simulink model "BasicAudio_TranslationEngine64"  (R2022b)
settings: Solver=FixedStepDiscrete  StartTime=0.0  StopTime=5  RelTol=1e-3  EnableMultiTasking=on
InitFcn:
  | % Initialize model
  | run([ ModelRootName() 'Init.m' ]);
  | 
  | % load library data
  | GainLibrary_data;
  | % Load saved values from partition process
  | CapturedConstMask.LoadMapFromFile(bdroot)
model workspace (MAT data in the model file):
  PreampVolumeTable_Idx : Simulink.Signal (value not decoded)
  Range : Simulink.Signal (value not decoded)
  Table_Idx : Simulink.Signal (value not decoded)
undefined symbols (not defined in the file or in its folder): Row
libraries: TuneVar x50, TOP x27, FeaturePath x7, CapturedConstLib x3
(part 3 of 4)

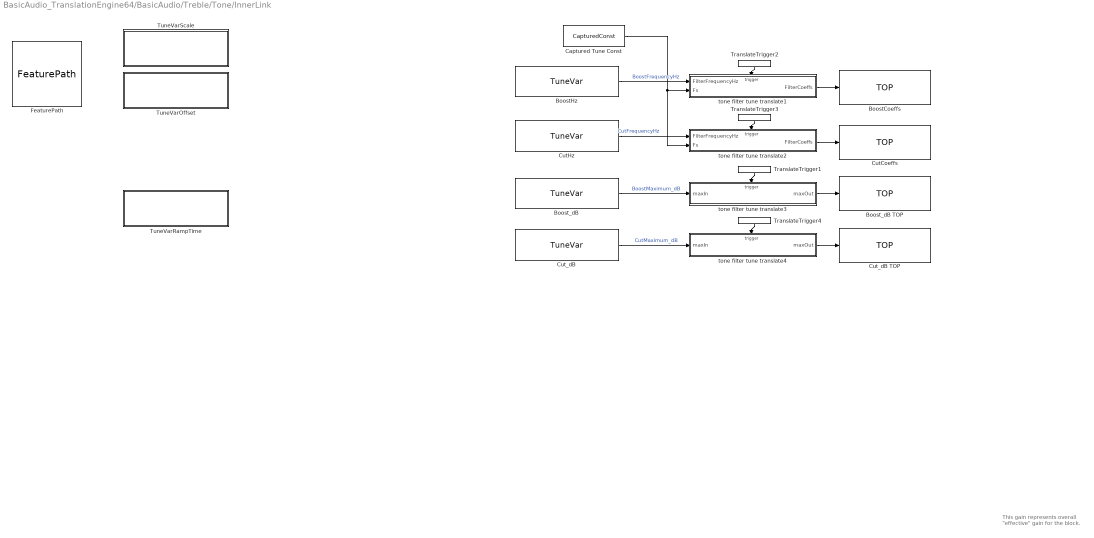
== system BasicAudio_TranslationEngine64/BasicAudio/Treble/Tone/InnerLink ==
  note: This gain represents overall
      | "effective" gain for the block.
  BoostCoeffs : TOP/TOP  TriggerInit=[-490 -218 -340 -162]  TopName=BoostCoeffs  DataTypeOut=single  BankNumber=Config.BankNumber  PreOverlay=false  PostOverlay=false  CompatibilityString=[]  Role=Automatic
      settings: SourceProductName=Bose Talaria
  BoostHz : TuneVar/TuneVar  Description=Indicates the 'corner frequency' of the target frequency band for the 'Boost' filter.  TuneName=BoostFrequencyHz  SpecifyMaxSize=off  VariableDim=1 (Row)  MaxSize=[1 1]  TunabilityNumber=1  MinValue=[]  MaxValue=[]  TriggerInit=[-1025 -225 -855 -175]  MaskValue=Config.DefaultBoostHz
      settings: SourceProductName=Bose Talaria
  Boost_dB : TuneVar/TuneVar  Description=Indicates the maximum impact in dB for the tone boost. This value must be positive. A negative boost impact would imply a gain cut instead!  TuneName=BoostMaximum_dB  SpecifyMaxSize=off  VariableDim=1 (Row)  MaxSize=[1 1]  TunabilityNumber=1  MinValue=[0]  MaxValue=[]  TriggerInit=[-1025 -40 -855 10]  MaskValue=Config.DefaultBoostDb
      settings: SourceProductName=Bose Talaria
  Boost_dB TOP : TOP/TOP  TriggerInit=[-490 -43 -340 13]  TopName=BoostMaximum_dB  DataTypeOut=single  BankNumber=Config.BankNumber  PreOverlay=false  PostOverlay=false  CompatibilityString=[]  Role=Automatic
      settings: SourceProductName=Bose Talaria
  Captured Tune Const : CapturedConstLib/CapturedConst  TriggerInit=[-945 -293 -845 -257]  Role=Automatic
      settings: SourceProductName=Bose Talaria
  CutCoeffs : TOP/TOP  TriggerInit=[-490 -128 -340 -72]  TopName=CutCoeffs  DataTypeOut=single  BankNumber=Config.BankNumber  PreOverlay=false  PostOverlay=false  CompatibilityString=[]  Role=Automatic
      settings: SourceProductName=Bose Talaria
  CutHz : TuneVar/TuneVar  Description=Indicates the 'corner frequency' of the target frequency band for the 'Cut' filter.  TuneName=CutFrequencyHz  SpecifyMaxSize=off  VariableDim=1 (Row)  MaxSize=[1 1]  TunabilityNumber=1  MinValue=[]  MaxValue=[]  TriggerInit=[-1025 -135 -855 -85]  MaskValue=Config.DefaultCutHz
      settings: SourceProductName=Bose Talaria
  Cut_dB : TuneVar/TuneVar  Description=Indicates the maximum impact in dB for the tone cut. This value must be positive. A negative cut impact would imply a gain boost instead!  TuneName=CutMaximum_dB  SpecifyMaxSize=off  VariableDim=1 (Row)  MaxSize=[1 1]  TunabilityNumber=1  MinValue=[0]  MaxValue=[]  TriggerInit=[-1025 45 -855 95]  MaskValue=Config.DefaultCutDb
      settings: SourceProductName=Bose Talaria
  Cut_dB TOP : TOP/TOP  TriggerInit=[-490 42 -340 98]  TopName=CutMaximum_dB  DataTypeOut=single  BankNumber=Config.BankNumber  PreOverlay=false  PostOverlay=false  CompatibilityString=[]  Role=Automatic
      settings: SourceProductName=Bose Talaria
  FeaturePath : FeaturePath/FeaturePath  FeatureName=Treble  IsGroup=off  GroupNumber=-1  IsModule=off  TriggerInit=[-1855 -266 -1740 -159]
      settings: SourceProductName=Bose Talaria
  TranslateTrigger1 : TuneVar/TranslateTrigger  TriggerInit=[-657 -60 -603 -50]
      settings: SourceProductName=Bose Talaria
  TranslateTrigger2 : TuneVar/TranslateTrigger  TriggerInit=[-657 -235 -603 -225]
      settings: SourceProductName=Bose Talaria
  TranslateTrigger3 : TuneVar/TranslateTrigger  TriggerInit=[-657 -145 -603 -135]
      settings: SourceProductName=Bose Talaria
  TranslateTrigger4 : TuneVar/TranslateTrigger  TriggerInit=[-657 25 -603 35]
      settings: SourceProductName=Bose Talaria
  TuneVarOffset : Subsystem  Description=Offset represents the midpoint of the index range, which separates the 'boost' indices from the 'cut' indices.  mask(Talaria Trivial Tune TOP){TriggerInit=[-1670 -213 -1500 -157], TopName=Offset, TuneName=Offset, DataTypeOut=single, MaskValue=Config.DefaultOffset, TunabilityNumber=1, MinValue=[], MaxValue=[], BankNumber=Config.BankNumber, PreOverlay=false, PostOverlay=false, UseSameName=on}
      mask prompts: TriggerInit "Hidden: MoveFcn redraw"; TopName "Name:"; TuneName "Name of TuneVar:"; DataTypeOut "Data type:"; MaskValue "Default Value:"; TunabilityNumber "Tunability:"; MinValue "Min Value:"; MaxValue "Max Value:"; BankNumber "Target memory bank number:"; PreOverlay "Requires pre-overlay action:"; PostOverlay "Requires post-overlay action:"; UseSameName "Use same name for tune variable and TOP"
      mask help: The TuneTOP block encapsultes a Target Overlay Parameter, a Tune Variable, and a Trivial Translation between them.
      mask init:
      | [ok,activeTopPath,activeTunePath] = TuneTOP_Mask.Init(gcbh);
      settings: MoveFcn=TuneTOP_Mask.CB_TriggerInit(gcbh);
      mask Callback TriggerInit: TuneTOP_Mask.CB_TriggerInit(gcbh);
      mask TypeOptions TopName: TOP/TopName
      mask TypeOptions TuneName: Tune Variable/TuneName
      mask TypeOptions DataTypeOut: TOP/DataTypeOut
      mask TypeOptions MaskValue: Tune Variable/MaskValue
      mask TypeOptions TunabilityNumber: Tune Variable/TunabilityNumber
      mask Callback TunabilityNumber: TuneVarMask.CB_TunabilityNumber(gcbh);
      mask TypeOptions MinValue: Tune Variable/MinValue
      mask TypeOptions MaxValue: Tune Variable/MaxValue
      mask TypeOptions BankNumber: TOP/BankNumber
      mask TypeOptions PreOverlay: TOP/PreOverlay
      mask TypeOptions PostOverlay: TOP/PostOverlay
      mask Callback UseSameName: TuneTOP_Mask.CB_UseSameName(gcbh);
      mask DialogControl toolPanel Prompt: Tuning Tool Hints
      mask DialogControl DescriptionGroup Prompt: Description
      mask DialogControl EditDescription Prompt: Edit Description
      mask DialogControl EditDescription Callback: TuneTOP_Mask.CB_EditDescription(gcbh);
      mask DialogControl TunabilityText Prompt: Easy: Changes nearly every tuning.
      mask DialogControl AdvancedPanel Prompt: Advanced
      mask DialogControl ConvertToFullTranslation Prompt: Irreversible conversion to full translation
      mask DialogControl ConvertToFullTranslation Callback: TuneTOP_Mask.CB_ConvertToFullTranslation(gcbh);
      mask DialogControl ErrorContainer Prompt: Error Messages
      mask Display:
      | % retrieve icon definition
      | [path,w,h] = TuneTOP_Mask.Icon();
      | 
      | % retrieve the block's pixel size
      | pos = get(gcbh,'position');
      | bw = pos(3) - pos(1);
      | bh = pos(4) - pos(2);
      | 
      | % draw centered icon
      | xAdj = bw/2 - w/2 + 5;
      | yAdj = bh/2 - h/2 + 4;
      | for i=1:length(path)
      | 	patch(path(i).x+xAdj, path(i).y+yAdj, path(i).rgb);
      | end
      | 
      | % show the top name or an X
      | if (exist('ok','var') && ok)
      | 	text(bw*0.5, bh*0.2, activeTopPath, 'horizontalAlignment', 'center');
      | 	patch(0,0,[1 1 1]);
      | 	patch(bw,bh,[1 1 1]);
      | else
      | 	tx=bw*0.03;
      | 	ty=bh*0.03;
      | 	patch([0 tx bw bw-tx], [ty 0 bh-ty bh], [1 0 0]);
      | 	patch([0 bw-tx bw tx], [bh-ty 0 ty bh], [1 0 0]);
      | end
  TuneVarRampTime : Subsystem  Description=This is the default ramp time that will be used if the RTC message has a '0' for both ramp time and ramp rate.  mask(Talaria Trivial Tune TOP){TriggerInit=[-1670 -18 -1500 38], TopName=ramptime, TuneName=ramptime, DataTypeOut=single, MaskValue=30, TunabilityNumber=1, MinValue=1, MaxValue=100000, BankNumber=0, PreOverlay=false, PostOverlay=false, UseSameName=on}
      mask prompts: TriggerInit "Hidden: MoveFcn redraw"; TopName "Name:"; TuneName "Name of TuneVar:"; DataTypeOut "Data type:"; MaskValue "Default Value:"; TunabilityNumber "Tunability:"; MinValue "Min Value:"; MaxValue "Max Value:"; BankNumber "Target memory bank number:"; PreOverlay "Requires pre-overlay action:"; PostOverlay "Requires post-overlay action:"; UseSameName "Use same name for tune variable and TOP"
      mask help: The TuneTOP block encapsultes a Target Overlay Parameter, a Tune Variable, and a Trivial Translation between them.
      mask init:
      | [ok,activeTopPath,activeTunePath] = TuneTOP_Mask.Init(gcbh);
      settings: MoveFcn=TuneTOP_Mask.CB_TriggerInit(gcbh);
      mask Callback TriggerInit: TuneTOP_Mask.CB_TriggerInit(gcbh);
      mask TypeOptions TopName: TOP/TopName
      mask TypeOptions TuneName: Tune Variable/TuneName
      mask TypeOptions DataTypeOut: TOP/DataTypeOut
      mask TypeOptions MaskValue: Tune Variable/MaskValue
      mask TypeOptions TunabilityNumber: Tune Variable/TunabilityNumber
      mask Callback TunabilityNumber: TuneVarMask.CB_TunabilityNumber(gcbh);
      mask TypeOptions MinValue: Tune Variable/MinValue
      mask TypeOptions MaxValue: Tune Variable/MaxValue
      mask TypeOptions BankNumber: TOP/BankNumber
      mask TypeOptions PreOverlay: TOP/PreOverlay
      mask TypeOptions PostOverlay: TOP/PostOverlay
      mask Callback UseSameName: TuneTOP_Mask.CB_UseSameName(gcbh);
      mask DialogControl toolPanel Prompt: Tuning Tool Hints
      mask DialogControl DescriptionGroup Prompt: Description
      mask DialogControl EditDescription Prompt: Edit Description
      mask DialogControl EditDescription Callback: TuneTOP_Mask.CB_EditDescription(gcbh);
      mask DialogControl TunabilityText Prompt: Easy: Changes nearly every tuning.
      mask DialogControl AdvancedPanel Prompt: Advanced
      mask DialogControl ConvertToFullTranslation Prompt: Irreversible conversion to full translation
      mask DialogControl ConvertToFullTranslation Callback: TuneTOP_Mask.CB_ConvertToFullTranslation(gcbh);
      mask DialogControl ErrorContainer Prompt: Error Messages
      mask Display:
      | % retrieve icon definition
      | [path,w,h] = TuneTOP_Mask.Icon();
      | 
      | % retrieve the block's pixel size
      | pos = get(gcbh,'position');
      | bw = pos(3) - pos(1);
      | bh = pos(4) - pos(2);
      | 
      | % draw centered icon
      | xAdj = bw/2 - w/2 + 5;
      | yAdj = bh/2 - h/2 + 4;
      | for i=1:length(path)
      | 	patch(path(i).x+xAdj, path(i).y+yAdj, path(i).rgb);
      | end
      | 
      | % show the top name or an X
      | if (exist('ok','var') && ok)
      | 	text(bw*0.5, bh*0.2, activeTopPath, 'horizontalAlignment', 'center');
      | 	patch(0,0,[1 1 1]);
      | 	patch(bw,bh,[1 1 1]);
      | else
      | 	tx=bw*0.03;
      | 	ty=bh*0.03;
      | 	patch([0 tx bw bw-tx], [ty 0 bh-ty bh], [1 0 0]);
      | 	patch([0 bw-tx bw tx], [bh-ty 0 ty bh], [1 0 0]);
      | end
  TuneVarScale : Subsystem  Description=Scale is used to normalize the linear gain to a value between +/- 1. The range (0,1] represents a boost while the range [-1,0) represents a cut. We use the number of available indices in each range (mapped to gain values between [-1,1]) as the denominator for normalization, i.e. as the 'Scale'.  mask(Talaria Trivial Tune TOP){TriggerInit=[-1670 -283 -1500 -227], TopName=Scale, TuneName=Scale, DataTypeOut=single, MaskValue=Config.DefaultScale, TunabilityNumber=1, MinValue=[], MaxValue=[], BankNumber=Config.BankNumber, PreOverlay=false, PostOverlay=false, UseSameName=on}
      mask prompts: TriggerInit "Hidden: MoveFcn redraw"; TopName "Name:"; TuneName "Name of TuneVar:"; DataTypeOut "Data type:"; MaskValue "Default Value:"; TunabilityNumber "Tunability:"; MinValue "Min Value:"; MaxValue "Max Value:"; BankNumber "Target memory bank number:"; PreOverlay "Requires pre-overlay action:"; PostOverlay "Requires post-overlay action:"; UseSameName "Use same name for tune variable and TOP"
      mask help: The TuneTOP block encapsultes a Target Overlay Parameter, a Tune Variable, and a Trivial Translation between them.
      mask init:
      | [ok,activeTopPath,activeTunePath] = TuneTOP_Mask.Init(gcbh);
      settings: MoveFcn=TuneTOP_Mask.CB_TriggerInit(gcbh);
      mask Callback TriggerInit: TuneTOP_Mask.CB_TriggerInit(gcbh);
      mask TypeOptions TopName: TOP/TopName
      mask TypeOptions TuneName: Tune Variable/TuneName
      mask TypeOptions DataTypeOut: TOP/DataTypeOut
      mask TypeOptions MaskValue: Tune Variable/MaskValue
      mask TypeOptions TunabilityNumber: Tune Variable/TunabilityNumber
      mask Callback TunabilityNumber: TuneVarMask.CB_TunabilityNumber(gcbh);
      mask TypeOptions MinValue: Tune Variable/MinValue
      mask TypeOptions MaxValue: Tune Variable/MaxValue
      mask TypeOptions BankNumber: TOP/BankNumber
      mask TypeOptions PreOverlay: TOP/PreOverlay
      mask TypeOptions PostOverlay: TOP/PostOverlay
      mask Callback UseSameName: TuneTOP_Mask.CB_UseSameName(gcbh);
      mask DialogControl toolPanel Prompt: Tuning Tool Hints
      mask DialogControl DescriptionGroup Prompt: Description
      mask DialogControl EditDescription Prompt: Edit Description
      mask DialogControl EditDescription Callback: TuneTOP_Mask.CB_EditDescription(gcbh);
      mask DialogControl TunabilityText Prompt: Easy: Changes nearly every tuning.
      mask DialogControl AdvancedPanel Prompt: Advanced
      mask DialogControl ConvertToFullTranslation Prompt: Irreversible conversion to full translation
      mask DialogControl ConvertToFullTranslation Callback: TuneTOP_Mask.CB_ConvertToFullTranslation(gcbh);
      mask DialogControl ErrorContainer Prompt: Error Messages
      mask Display:
      | % retrieve icon definition
      | [path,w,h] = TuneTOP_Mask.Icon();
      | 
      | % retrieve the block's pixel size
      | pos = get(gcbh,'position');
      | bw = pos(3) - pos(1);
      | bh = pos(4) - pos(2);
      | 
      | % draw centered icon
      | xAdj = bw/2 - w/2 + 5;
      | yAdj = bh/2 - h/2 + 4;
      | for i=1:length(path)
      | 	patch(path(i).x+xAdj, path(i).y+yAdj, path(i).rgb);
      | end
      | 
      | % show the top name or an X
      | if (exist('ok','var') && ok)
      | 	text(bw*0.5, bh*0.2, activeTopPath, 'horizontalAlignment', 'center');
      | 	patch(0,0,[1 1 1]);
      | 	patch(bw,bh,[1 1 1]);
      | else
      | 	tx=bw*0.03;
      | 	ty=bh*0.03;
      | 	patch([0 tx bw bw-tx], [ty 0 bh-ty bh], [1 0 0]);
      | 	patch([0 bw-tx bw tx], [bh-ty 0 ty bh], [1 0 0]);
      | end
  tone filter tune translate1 : MATLAB Function  TreatAsAtomicUnit=on  mask{MaskFilterType=Config.FilterType}
      mask prompts: MaskFilterType "Filter type"
  tone filter tune translate2 : MATLAB Function  TreatAsAtomicUnit=on  mask{MaskFilterType=Config.FilterType}
      mask prompts: MaskFilterType "Filter type"
  tone filter tune translate3 : MATLAB Function  TreatAsAtomicUnit=on
  tone filter tune translate4 : MATLAB Function  TreatAsAtomicUnit=on
  wires:
  TranslateTrigger2/1 -> tone filter tune translate1/Trigger
  BoostHz/1 -> tone filter tune translate1/1(FilterFrequencyHz)  "BoostFrequencyHz"
  TranslateTrigger3/1 -> tone filter tune translate2/Trigger
  CutHz/1 -> tone filter tune translate2/1(FilterFrequencyHz)  "CutFrequencyHz"
  tone filter tune translate1/1(FilterCoeffs) -> BoostCoeffs/1
  tone filter tune translate2/1(FilterCoeffs) -> CutCoeffs/1
  Boost_dB/1 -> tone filter tune translate3/1(maxIn)  "BoostMaximum_dB"
  tone filter tune translate3/1(maxOut) -> Boost_dB TOP/1
  Cut_dB/1 -> tone filter tune translate4/1(maxIn)  "CutMaximum_dB"
  tone filter tune translate4/1(maxOut) -> Cut_dB TOP/1
  Captured Tune Const/1 -> tone filter tune translate2/2(Fs), tone filter tune translate1/2(Fs)
  TranslateTrigger1/1 -> tone filter tune translate3/Trigger
  TranslateTrigger4/1 -> tone filter tune translate4/Trigger

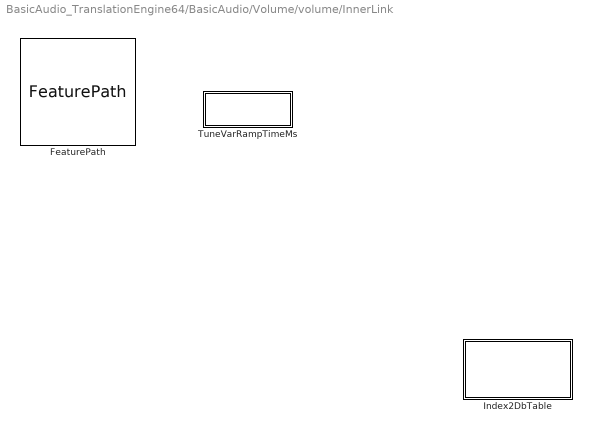
== system BasicAudio_TranslationEngine64/BasicAudio/Volume/volume/InnerLink ==
  FeaturePath : FeaturePath/FeaturePath  FeatureName=Volume  IsGroup=off  GroupNumber=-1  IsModule=off  TriggerInit=[640 269 755 376]
      settings: SourceProductName=Bose Talaria
  Index2DbTable : Subsystem  mask(Blocklib Index2DbTable){Config=Config}
      mask prompts: Config "Index2DbTableConfig"
      mask help: This block contains overlay tuning data for an index-to-dB lookup table. Provide the maximum number of points in the table as a build-time variable. The TuneVar is variable size, but must define at least two points (i.e. two rows, or four values).
      mask init:
      | blkh=gcbh;
      | Config=BTConfig.Assert(blkh,Config);
      | 
      | Config.Validate();
      mask Help:
      | This block contains overlay tuning data which defines an index-to-dB lookup table.
      | Each row of the tuning data contains an index and a dB value.
      | 
      | Tuning data
      | ---------------
      |    tune index: normalized value between 0 and 1
      |    tune value: dB value such as 0 (aka linear "1") or -100 (aka "very quiet")
      | 
      | Inports
      | ----------
      |    trigger: function call trigger that invokes the lookup from inport index to output dB
      |    index: an 8-bit integer index between [0:255] corresponding to the tuning index range [0:1]
      | 
      | Outport
      | -----------
      |    The resulting dB value looked up in the tuned table by using the inbound index
  TuneVarRampTimeMs : Subsystem  mask(Talaria Trivial Tune TOP){TriggerInit=[825 324 910 356], TopName=RampTime, TuneName=RampTime, DataTypeOut=single, MaskValue=100, TunabilityNumber=1, MinValue=[], MaxValue=[], BankNumber=0, PreOverlay=false, PostOverlay=false, UseSameName=on}
      mask prompts: TriggerInit "Hidden: MoveFcn redraw"; TopName "Name:"; TuneName "Name of TuneVar:"; DataTypeOut "Data type:"; MaskValue "Default Value:"; TunabilityNumber "Tunability:"; MinValue "Min Value:"; MaxValue "Max Value:"; BankNumber "Target memory bank number:"; PreOverlay "Requires pre-overlay action:"; PostOverlay "Requires post-overlay action:"; UseSameName "Use same name for tune variable and TOP"
      mask help: The TuneTOP block encapsultes a Target Overlay Parameter, a Tune Variable, and a Trivial Translation between them.
      mask init:
      | [ok,activeTopPath,activeTunePath] = TuneTOP_Mask.Init(gcbh);
      settings: MoveFcn=TuneTOP_Mask.CB_TriggerInit(gcbh);
      mask Callback TriggerInit: TuneTOP_Mask.CB_TriggerInit(gcbh);
      mask TypeOptions TopName: TOP/TopName
      mask TypeOptions TuneName: Tune Variable/TuneName
      mask TypeOptions DataTypeOut: TOP/DataTypeOut
      mask TypeOptions MaskValue: Tune Variable/MaskValue
      mask TypeOptions TunabilityNumber: Tune Variable/TunabilityNumber
      mask Callback TunabilityNumber: TuneVarMask.CB_TunabilityNumber(gcbh);
      mask TypeOptions MinValue: Tune Variable/MinValue
      mask TypeOptions MaxValue: Tune Variable/MaxValue
      mask TypeOptions BankNumber: TOP/BankNumber
      mask TypeOptions PreOverlay: TOP/PreOverlay
      mask TypeOptions PostOverlay: TOP/PostOverlay
      mask Callback UseSameName: TuneTOP_Mask.CB_UseSameName(gcbh);
      mask DialogControl toolPanel Prompt: Tuning Tool Hints
      mask DialogControl DescriptionGroup Prompt: Description
      mask DialogControl EditDescription Prompt: Edit Description
      mask DialogControl EditDescription Callback: TuneTOP_Mask.CB_EditDescription(gcbh);
      mask DialogControl TunabilityText Prompt: Easy: Changes nearly every tuning.
      mask DialogControl AdvancedPanel Prompt: Advanced
      mask DialogControl ConvertToFullTranslation Prompt: Irreversible conversion to full translation
      mask DialogControl ConvertToFullTranslation Callback: TuneTOP_Mask.CB_ConvertToFullTranslation(gcbh);
      mask DialogControl ErrorContainer Prompt: Error Messages
      mask DialogControl ErrorText Prompt: No overlay group found. Declare one in a FeaturePath.
      mask Display:
      | % retrieve icon definition
      | [path,w,h] = TuneTOP_Mask.Icon();
      | 
      | % retrieve the block's pixel size
      | pos = get(gcbh,'position');
      | bw = pos(3) - pos(1);
      | bh = pos(4) - pos(2);
      | 
      | % draw centered icon
      | xAdj = bw/2 - w/2 + 5;
      | yAdj = bh/2 - h/2 + 4;
      | for i=1:length(path)
      | 	patch(path(i).x+xAdj, path(i).y+yAdj, path(i).rgb);
      | end
      | 
      | % show the top name or an X
      | if (exist('ok','var') && ok)
      | 	text(bw*0.5, bh*0.2, activeTopPath, 'horizontalAlignment', 'center');
      | 	patch(0,0,[1 1 1]);
      | 	patch(bw,bh,[1 1 1]);
      | else
      | 	tx=bw*0.03;
      | 	ty=bh*0.03;
      | 	patch([0 tx bw bw-tx], [ty 0 bh-ty bh], [1 0 0]);
      | 	patch([0 bw-tx bw tx], [bh-ty 0 ty bh], [1 0 0]);
      | end

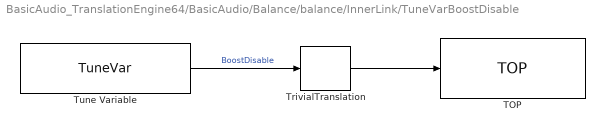
== system BasicAudio_TranslationEngine64/BasicAudio/Balance/balance/InnerLink/TuneVarBoostDisable ==
  TOP : TOP/TOP  TriggerInit=[440 20 585 80]  TopName=BoostDisable  DataTypeOut=single  BankNumber=BankNumber  PreOverlay=PreOverlay  PostOverlay=PostOverlay  CompatibilityString=[]  Role=Automatic
      settings: SourceProductName=Bose Talaria
  TrivialTranslation : TuneVar/TrivialTranslation  TriggerInit=[300 28 350 72]
      settings: SourceProductName=Bose Talaria
  Tune Variable : TuneVar/TuneVar  TuneName=BoostDisable  SpecifyMaxSize=off  VariableDim=1 (Row)  MaxSize=[1 1]  TunabilityNumber=2  MinValue=MinValue  MaxValue=MaxValue  TriggerInit=[20 25 190 75]  MaskValue=MaskValue
      settings: SourceProductName=Bose Talaria
  wires:
  Tune Variable/1 -> TrivialTranslation/1  "BoostDisable"
  TrivialTranslation/1 -> TOP/1

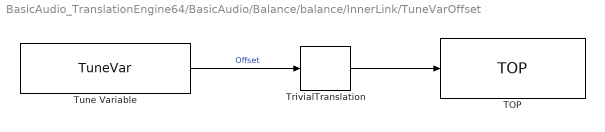
== system BasicAudio_TranslationEngine64/BasicAudio/Balance/balance/InnerLink/TuneVarOffset ==
  TOP : TOP/TOP  TriggerInit=[440 20 585 80]  TopName=Offset  DataTypeOut=single  BankNumber=BankNumber  PreOverlay=PreOverlay  PostOverlay=PostOverlay  CompatibilityString=[]  Role=Automatic
      settings: SourceProductName=Bose Talaria
  TrivialTranslation : TuneVar/TrivialTranslation  TriggerInit=[300 28 350 72]
      settings: SourceProductName=Bose Talaria
  Tune Variable : TuneVar/TuneVar  TuneName=Offset  SpecifyMaxSize=off  VariableDim=1 (Row)  MaxSize=[1 1]  TunabilityNumber=3  MinValue=MinValue  MaxValue=MaxValue  TriggerInit=[20 25 190 75]  MaskValue=MaskValue
      settings: SourceProductName=Bose Talaria
  wires:
  Tune Variable/1 -> TrivialTranslation/1  "Offset"
  TrivialTranslation/1 -> TOP/1

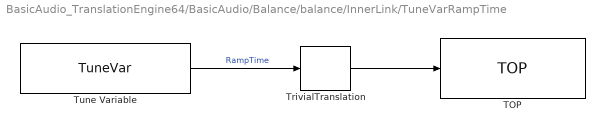
== system BasicAudio_TranslationEngine64/BasicAudio/Balance/balance/InnerLink/TuneVarRampTime ==
  TOP : TOP/TOP  TriggerInit=[440 20 585 80]  TopName=RampTime  DataTypeOut=single  BankNumber=BankNumber  PreOverlay=PreOverlay  PostOverlay=PostOverlay  CompatibilityString=[]  Role=Automatic
      settings: SourceProductName=Bose Talaria
  TrivialTranslation : TuneVar/TrivialTranslation  TriggerInit=[300 28 350 72]
      settings: SourceProductName=Bose Talaria
  Tune Variable : TuneVar/TuneVar  TuneName=RampTime  SpecifyMaxSize=off  VariableDim=1 (Row)  MaxSize=[1 1]  TunabilityNumber=2  MinValue=MinValue  MaxValue=MaxValue  TriggerInit=[20 25 190 75]  MaskValue=MaskValue
      settings: SourceProductName=Bose Talaria
  wires:
  Tune Variable/1 -> TrivialTranslation/1  "RampTime"
  TrivialTranslation/1 -> TOP/1

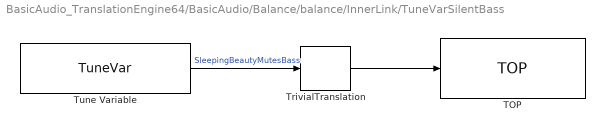
== system BasicAudio_TranslationEngine64/BasicAudio/Balance/balance/InnerLink/TuneVarSilentBass ==
  TOP : TOP/TOP  TriggerInit=[440 20 585 80]  TopName=SleepingBeautyMutesBass  DataTypeOut=single  BankNumber=BankNumber  PreOverlay=PreOverlay  PostOverlay=PostOverlay  CompatibilityString=[]  Role=Automatic
      settings: SourceProductName=Bose Talaria
  TrivialTranslation : TuneVar/TrivialTranslation  TriggerInit=[300 28 350 72]
      settings: SourceProductName=Bose Talaria
  Tune Variable : TuneVar/TuneVar  TuneName=SleepingBeautyMutesBass  SpecifyMaxSize=off  VariableDim=1 (Row)  MaxSize=[1 1]  TunabilityNumber=1  MinValue=MinValue  MaxValue=MaxValue  TriggerInit=[20 25 190 75]  MaskValue=MaskValue
      settings: SourceProductName=Bose Talaria
  wires:
  Tune Variable/1 -> TrivialTranslation/1  "SleepingBeautyMutesBass"
  TrivialTranslation/1 -> TOP/1

== system BasicAudio_TranslationEngine64/BasicAudio/Balance/balance/InnerLink/TuneVarSilentExtreme ==
  TOP : TOP/TOP  TriggerInit=[440 20 585 80]  TopName=EnableSilentExtreme  DataTypeOut=single  BankNumber=BankNumber  PreOverlay=PreOverlay  PostOverlay=PostOverlay  CompatibilityString=[]  Role=Automatic
      settings: SourceProductName=Bose Talaria
  TrivialTranslation : TuneVar/TrivialTranslation  TriggerInit=[300 28 350 72]
      settings: SourceProductName=Bose Talaria
  Tune Variable : TuneVar/TuneVar  TuneName=EnableSilentExtreme  SpecifyMaxSize=off  VariableDim=1 (Row)  MaxSize=[1 1]  TunabilityNumber=2  MinValue=MinValue  MaxValue=MaxValue  TriggerInit=[20 25 190 75]  MaskValue=MaskValue
      settings: SourceProductName=Bose Talaria
  wires:
  Tune Variable/1 -> TrivialTranslation/1  "EnableSilentExtreme"
  TrivialTranslation/1 -> TOP/1

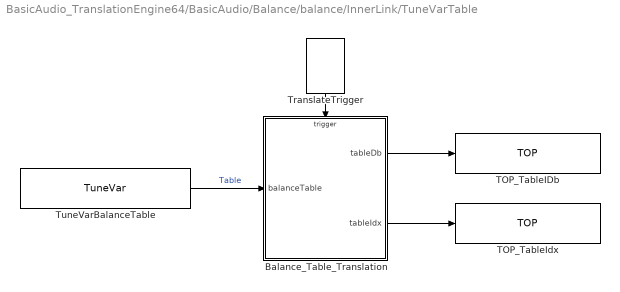
== system BasicAudio_TranslationEngine64/BasicAudio/Balance/balance/InnerLink/TuneVarTable ==
  Balance_Table_Translation : MATLAB Function  TreatAsAtomicUnit=on
  TOP_TableIDb : TOP/TOP  TriggerInit=[455 -5 600 35]  TopName=TableDb  DataTypeOut=single  BankNumber=0  PreOverlay=false  PostOverlay=false  CompatibilityString=[]  Role=Automatic
      settings: SourceProductName=Bose Talaria
  TOP_TableIdx : TOP/TOP  TriggerInit=[455 65 600 105]  TopName=TableIdx  DataTypeOut=single  BankNumber=Config.BankNumber  PreOverlay=false  PostOverlay=false  CompatibilityString=[]  Role=Automatic
      settings: SourceProductName=Bose Talaria
  TranslateTrigger : TuneVar/TranslateTrigger  TriggerInit=[306 -100 344 -45]
      settings: SourceProductName=Bose Talaria
  TuneVarBalanceTable : TuneVar/TuneVar  Description=Define the balance curve using a table, with the first column being the list of indices and the second column being the corresponding balance gains in dB. Gain values for indices in between the elements in the table are linearly interpolated.  TuneName=Table  SpecifyMaxSize=on  VariableDim=1 (Row)  MaxSize=[30 2]  TunabilityNumber=3  MinValue=0  MaxValue=[]  TriggerInit=[20 30 190 70]  MaskValue=[[0,10,31,52,74,95,116,128,138,159,180,202,223,244,255];[-30,-27,-14,-7,-5,-3,-1,0,-1,-3,-5,-7,-14,-27,-30]]'
      settings: SourceProductName=Bose Talaria
  wires:
  Balance_Table_Translation/1(tableDb) -> TOP_TableIDb/1
  TranslateTrigger/1 -> Balance_Table_Translation/Trigger
  Balance_Table_Translation/2(tableIdx) -> TOP_TableIdx/1
  TuneVarBalanceTable/1 -> Balance_Table_Translation/1(balanceTable)  "Table"

== system BasicAudio_TranslationEngine64/BasicAudio/Bass/Tone/InnerLink/TuneVarOffset ==
  TOP : TOP/TOP  TriggerInit=[440 20 585 80]  TopName=Offset  DataTypeOut=single  BankNumber=BankNumber  PreOverlay=PreOverlay  PostOverlay=PostOverlay  CompatibilityString=[]  Role=Automatic
      settings: SourceProductName=Bose Talaria
  TrivialTranslation : TuneVar/TrivialTranslation  TriggerInit=[300 28 350 72]
      settings: SourceProductName=Bose Talaria
  Tune Variable : TuneVar/TuneVar  TuneName=Offset  SpecifyMaxSize=off  VariableDim=1 (Row)  MaxSize=[1 1]  TunabilityNumber=1  MinValue=MinValue  MaxValue=MaxValue  TriggerInit=[20 25 190 75]  MaskValue=MaskValue
      settings: SourceProductName=Bose Talaria
  wires:
  Tune Variable/1 -> TrivialTranslation/1  "Offset"
  TrivialTranslation/1 -> TOP/1

== system BasicAudio_TranslationEngine64/BasicAudio/Bass/Tone/InnerLink/TuneVarRampTime ==
  TOP : TOP/TOP  TriggerInit=[440 20 585 80]  TopName=ramptime  DataTypeOut=single  BankNumber=BankNumber  PreOverlay=PreOverlay  PostOverlay=PostOverlay  CompatibilityString=[]  Role=Automatic
      settings: SourceProductName=Bose Talaria
  TrivialTranslation : TuneVar/TrivialTranslation  TriggerInit=[300 28 350 72]
      settings: SourceProductName=Bose Talaria
  Tune Variable : TuneVar/TuneVar  TuneName=ramptime  SpecifyMaxSize=off  VariableDim=1 (Row)  MaxSize=[1 1]  TunabilityNumber=1  MinValue=MinValue  MaxValue=MaxValue  TriggerInit=[20 25 190 75]  MaskValue=MaskValue
      settings: SourceProductName=Bose Talaria
  wires:
  Tune Variable/1 -> TrivialTranslation/1  "ramptime"
  TrivialTranslation/1 -> TOP/1

== system BasicAudio_TranslationEngine64/BasicAudio/Bass/Tone/InnerLink/TuneVarScale ==
  TOP : TOP/TOP  TriggerInit=[440 20 585 80]  TopName=Scale  DataTypeOut=single  BankNumber=BankNumber  PreOverlay=PreOverlay  PostOverlay=PostOverlay  CompatibilityString=[]  Role=Automatic
      settings: SourceProductName=Bose Talaria
  TrivialTranslation : TuneVar/TrivialTranslation  TriggerInit=[300 28 350 72]
      settings: SourceProductName=Bose Talaria
  Tune Variable : TuneVar/TuneVar  TuneName=Scale  SpecifyMaxSize=off  VariableDim=1 (Row)  MaxSize=[1 1]  TunabilityNumber=1  MinValue=MinValue  MaxValue=MaxValue  TriggerInit=[20 25 190 75]  MaskValue=MaskValue
      settings: SourceProductName=Bose Talaria
  wires:
  Tune Variable/1 -> TrivialTranslation/1  "Scale"
  TrivialTranslation/1 -> TOP/1

== system BasicAudio_TranslationEngine64/BasicAudio/Mute/mute/InnerLink/MuteControl ==
  FeaturePath : FeaturePath/FeaturePath  FeatureName=Mute  IsGroup=off  GroupNumber=-1  IsModule=off  TriggerInit=[180 39 295 146]
      settings: SourceProductName=Bose Talaria
  TuneVarRampTime : Subsystem  Description=|  mask(Talaria Trivial Tune TOP){TriggerInit=[295 232 465 288], TopName=RampTime, TuneName=RampTime, DataTypeOut=single, MaskValue=Config.DefaultRampTimeMsec, TunabilityNumber=1, MinValue=1, MaxValue=100000, BankNumber=0, PreOverlay=false, PostOverlay=false, UseSameName=on}
      | Specifies the default value of ramp time for the Mute or Unmute operation.
      | Used only when the RTC message does not contain either ramp rate or ramp time.
      mask prompts: TriggerInit "Hidden: MoveFcn redraw"; TopName "Name:"; TuneName "Name of TuneVar:"; DataTypeOut "Data type:"; MaskValue "Default Value:"; TunabilityNumber "Tunability:"; MinValue "Min Value:"; MaxValue "Max Value:"; BankNumber "Target memory bank number:"; PreOverlay "Requires pre-overlay action:"; PostOverlay "Requires post-overlay action:"; UseSameName "Use same name for tune variable and TOP"
      mask help: The TuneTOP block encapsultes a Target Overlay Parameter, a Tune Variable, and a Trivial Translation between them.
      mask init:
      | [ok,activeTopPath,activeTunePath] = TuneTOP_Mask.Init(gcbh);
      settings: MoveFcn=TuneTOP_Mask.CB_TriggerInit(gcbh);
      mask Callback TriggerInit: TuneTOP_Mask.CB_TriggerInit(gcbh);
      mask TypeOptions TopName: TOP/TopName
      mask TypeOptions TuneName: Tune Variable/TuneName
      mask TypeOptions DataTypeOut: TOP/DataTypeOut
      mask TypeOptions MaskValue: Tune Variable/MaskValue
      mask TypeOptions TunabilityNumber: Tune Variable/TunabilityNumber
      mask Callback TunabilityNumber: TuneVarMask.CB_TunabilityNumber(gcbh);
      mask TypeOptions MinValue: Tune Variable/MinValue
      mask TypeOptions MaxValue: Tune Variable/MaxValue
      mask TypeOptions BankNumber: TOP/BankNumber
      mask TypeOptions PreOverlay: TOP/PreOverlay
      mask TypeOptions PostOverlay: TOP/PostOverlay
      mask Callback UseSameName: TuneTOP_Mask.CB_UseSameName(gcbh);
      mask DialogControl toolPanel Prompt: Tuning Tool Hints
      mask DialogControl DescriptionGroup Prompt: Description
      mask DialogControl EditDescription Prompt: Edit Description
      mask DialogControl EditDescription Callback: TuneTOP_Mask.CB_EditDescription(gcbh);
      mask DialogControl TunabilityText Prompt: Easy: Changes nearly every tuning.
      mask DialogControl AdvancedPanel Prompt: Advanced
      mask DialogControl ConvertToFullTranslation Prompt: Irreversible conversion to full translation
      mask DialogControl ConvertToFullTranslation Callback: TuneTOP_Mask.CB_ConvertToFullTranslation(gcbh);
      mask DialogControl ErrorContainer Prompt: Error Messages
      mask Display:
      | % retrieve icon definition
      | [path,w,h] = TuneTOP_Mask.Icon();
      | 
      | % retrieve the block's pixel size
      | pos = get(gcbh,'position');
      | bw = pos(3) - pos(1);
      | bh = pos(4) - pos(2);
      | 
      | % draw centered icon
      | xAdj = bw/2 - w/2 + 5;
      | yAdj = bh/2 - h/2 + 4;
      | for i=1:length(path)
      | 	patch(path(i).x+xAdj, path(i).y+yAdj, path(i).rgb);
      | end
      | 
      | % show the top name or an X
      | if (exist('ok','var') && ok)
      | 	text(bw*0.5, bh*0.2, activeTopPath, 'horizontalAlignment', 'center');
      | 	patch(0,0,[1 1 1]);
      | 	patch(bw,bh,[1 1 1]);
      | else
      | 	tx=bw*0.03;
      | 	ty=bh*0.03;
      | 	patch([0 tx bw bw-tx], [ty 0 bh-ty bh], [1 0 0]);
      | 	patch([0 bw-tx bw tx], [bh-ty 0 ty bh], [1 0 0]);
      | end

== system BasicAudio_TranslationEngine64/BasicAudio/Treble/Tone/InnerLink/TuneVarOffset ==
  TOP : TOP/TOP  TriggerInit=[440 20 585 80]  TopName=Offset  DataTypeOut=single  BankNumber=BankNumber  PreOverlay=PreOverlay  PostOverlay=PostOverlay  CompatibilityString=[]  Role=Automatic
      settings: SourceProductName=Bose Talaria
  TrivialTranslation : TuneVar/TrivialTranslation  TriggerInit=[300 28 350 72]
      settings: SourceProductName=Bose Talaria
  Tune Variable : TuneVar/TuneVar  TuneName=Offset  SpecifyMaxSize=off  VariableDim=1 (Row)  MaxSize=[1 1]  TunabilityNumber=1  MinValue=MinValue  MaxValue=MaxValue  TriggerInit=[20 25 190 75]  MaskValue=MaskValue
      settings: SourceProductName=Bose Talaria
  wires:
  Tune Variable/1 -> TrivialTranslation/1  "Offset"
  TrivialTranslation/1 -> TOP/1

== system BasicAudio_TranslationEngine64/BasicAudio/Treble/Tone/InnerLink/TuneVarRampTime ==
  TOP : TOP/TOP  TriggerInit=[440 20 585 80]  TopName=ramptime  DataTypeOut=single  BankNumber=BankNumber  PreOverlay=PreOverlay  PostOverlay=PostOverlay  CompatibilityString=[]  Role=Automatic
      settings: SourceProductName=Bose Talaria
  TrivialTranslation : TuneVar/TrivialTranslation  TriggerInit=[300 28 350 72]
      settings: SourceProductName=Bose Talaria
  Tune Variable : TuneVar/TuneVar  TuneName=ramptime  SpecifyMaxSize=off  VariableDim=1 (Row)  MaxSize=[1 1]  TunabilityNumber=1  MinValue=MinValue  MaxValue=MaxValue  TriggerInit=[20 25 190 75]  MaskValue=MaskValue
      settings: SourceProductName=Bose Talaria
  wires:
  Tune Variable/1 -> TrivialTranslation/1  "ramptime"
  TrivialTranslation/1 -> TOP/1

== system BasicAudio_TranslationEngine64/BasicAudio/Treble/Tone/InnerLink/TuneVarScale ==
  TOP : TOP/TOP  TriggerInit=[440 20 585 80]  TopName=Scale  DataTypeOut=single  BankNumber=BankNumber  PreOverlay=PreOverlay  PostOverlay=PostOverlay  CompatibilityString=[]  Role=Automatic
      settings: SourceProductName=Bose Talaria
  TrivialTranslation : TuneVar/TrivialTranslation  TriggerInit=[300 28 350 72]
      settings: SourceProductName=Bose Talaria
  Tune Variable : TuneVar/TuneVar  TuneName=Scale  SpecifyMaxSize=off  VariableDim=1 (Row)  MaxSize=[1 1]  TunabilityNumber=1  MinValue=MinValue  MaxValue=MaxValue  TriggerInit=[20 25 190 75]  MaskValue=MaskValue
      settings: SourceProductName=Bose Talaria
  wires:
  Tune Variable/1 -> TrivialTranslation/1  "Scale"
  TrivialTranslation/1 -> TOP/1

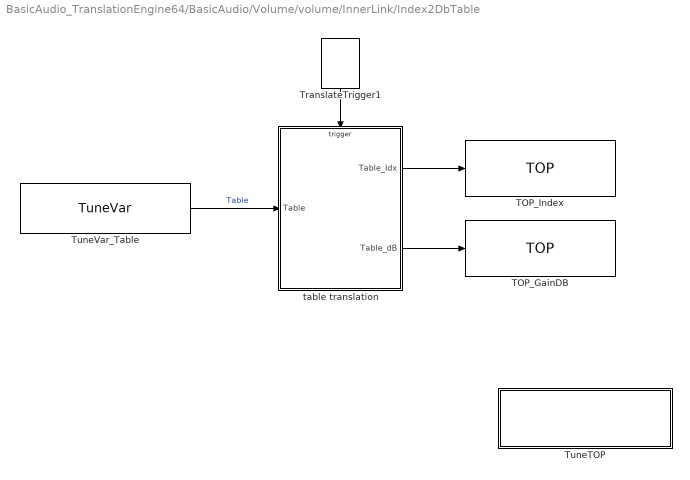
== system BasicAudio_TranslationEngine64/BasicAudio/Volume/volume/InnerLink/Index2DbTable ==
  TOP_GainDB : TOP/TOP  TriggerInit=[635 177 785 233]  TopName=Table_dB  DataTypeOut=Inherit: Same as input  BankNumber=Config.BankNumber  PreOverlay=false  PostOverlay=false  CompatibilityString=[]  Role=Automatic
      settings: SourceProductName=Bose Talaria
  TOP_Index : TOP/TOP  TriggerInit=[635 97 785 153]  TopName=Table_Idx  DataTypeOut=Inherit: Same as input  BankNumber=Config.BankNumber  PreOverlay=false  PostOverlay=false  CompatibilityString=[]  Role=Automatic
      settings: SourceProductName=Bose Talaria
  TranslateTrigger1 : TuneVar/TranslateTrigger  TriggerInit=[491 -5 529 45]
      settings: SourceProductName=Bose Talaria
  TuneTOP : Subsystem  Description=Variable limits the maximum *dB offset* which will be applied to the gain as part of table lookup. It does *not* directly impact the maximum gain applied, only the maximum dB offset.  mask(Talaria Trivial Tune TOP){TriggerInit=[670 347 840 403], TopName=maxgain, TuneName=maxgain, DataTypeOut=single, MaskValue=Config.DefaultMaxDbOffset, TunabilityNumber=1, MinValue=[], MaxValue=[], BankNumber=0, PreOverlay=false, PostOverlay=false, UseSameName=on}
      mask prompts: TriggerInit "Hidden: MoveFcn redraw"; TopName "Name:"; TuneName "Name of TuneVar:"; DataTypeOut "Data type:"; MaskValue "Default Value:"; TunabilityNumber "Tunability:"; MinValue "Min Value:"; MaxValue "Max Value:"; BankNumber "Target memory bank number:"; PreOverlay "Requires pre-overlay action:"; PostOverlay "Requires post-overlay action:"; UseSameName "Use same name for tune variable and TOP"
      mask help: The TuneTOP block encapsultes a Target Overlay Parameter, a Tune Variable, and a Trivial Translation between them.
      mask init:
      | [ok,activeTopPath,activeTunePath] = TuneTOP_Mask.Init(gcbh);
      settings: MoveFcn=TuneTOP_Mask.CB_TriggerInit(gcbh);
      mask Callback TriggerInit: TuneTOP_Mask.CB_TriggerInit(gcbh);
      mask TypeOptions TopName: TOP/TopName
      mask TypeOptions TuneName: Tune Variable/TuneName
      mask TypeOptions DataTypeOut: TOP/DataTypeOut
      mask TypeOptions MaskValue: Tune Variable/MaskValue
      mask TypeOptions TunabilityNumber: Tune Variable/TunabilityNumber
      mask Callback TunabilityNumber: TuneVarMask.CB_TunabilityNumber(gcbh);
      mask TypeOptions MinValue: Tune Variable/MinValue
      mask TypeOptions MaxValue: Tune Variable/MaxValue
      mask TypeOptions BankNumber: TOP/BankNumber
      mask TypeOptions PreOverlay: TOP/PreOverlay
      mask TypeOptions PostOverlay: TOP/PostOverlay
      mask Callback UseSameName: TuneTOP_Mask.CB_UseSameName(gcbh);
      mask DialogControl toolPanel Prompt: Tuning Tool Hints
      mask DialogControl DescriptionGroup Prompt: Description
      mask DialogControl EditDescription Prompt: Edit Description
      mask DialogControl EditDescription Callback: TuneTOP_Mask.CB_EditDescription(gcbh);
      mask DialogControl TunabilityText Prompt: Easy: Changes nearly every tuning.
      mask DialogControl AdvancedPanel Prompt: Advanced
      mask DialogControl ConvertToFullTranslation Prompt: Irreversible conversion to full translation
      mask DialogControl ConvertToFullTranslation Callback: TuneTOP_Mask.CB_ConvertToFullTranslation(gcbh);
      mask DialogControl ErrorContainer Prompt: Error Messages
      mask Display:
      | % retrieve icon definition
      | [path,w,h] = TuneTOP_Mask.Icon();
      | 
      | % retrieve the block's pixel size
      | pos = get(gcbh,'position');
      | bw = pos(3) - pos(1);
      | bh = pos(4) - pos(2);
      | 
      | % draw centered icon
      | xAdj = bw/2 - w/2 + 5;
      | yAdj = bh/2 - h/2 + 4;
      | for i=1:length(path)
      | 	patch(path(i).x+xAdj, path(i).y+yAdj, path(i).rgb);
      | end
      | 
      | % show the top name or an X
      | if (exist('ok','var') && ok)
      | 	text(bw*0.5, bh*0.2, activeTopPath, 'horizontalAlignment', 'center');
      | 	patch(0,0,[1 1 1]);
      | 	patch(bw,bh,[1 1 1]);
      | else
      | 	tx=bw*0.03;
      | 	ty=bh*0.03;
      | 	patch([0 tx bw bw-tx], [ty 0 bh-ty bh], [1 0 0]);
      | 	patch([0 bw-tx bw tx], [bh-ty 0 ty bh], [1 0 0]);
      | end
  TuneVar_Table : TuneVar/TuneVar  Description=|  TuneName=Table  SpecifyMaxSize=on  VariableDim=1 (Row)  MaxSize=[Config.MaximumTablePoints 2]  TunabilityNumber=2  MinValue=[0;-100]  MaxValue=[1;0]  TriggerInit=[190 140 360 190]  MaskValue=Config.DefaultTable
      | <HTML>Gain table maps index to gain.
      | The index values are <FONT color="red">normalized</Font> floats between 0 and 1 while the gains are in dB (i.e. 0 implies no attenuation).
      | </html>
      settings: SourceProductName=Bose Talaria
  table translation : MATLAB Function  TreatAsAtomicUnit=on
  wires:
  TuneVar_Table/1 -> table translation/1(Table)  "Table"
  TranslateTrigger1/1 -> table translation/Trigger
  table translation/1(Table_Idx) -> TOP_Index/1
  table translation/2(Table_dB) -> TOP_GainDB/1

== system BasicAudio_TranslationEngine64/BasicAudio/Volume/volume/InnerLink/TuneVarRampTimeMs ==
  TOP : TOP/TOP  TriggerInit=[440 20 585 80]  TopName=RampTime  DataTypeOut=single  BankNumber=BankNumber  PreOverlay=PreOverlay  PostOverlay=PostOverlay  CompatibilityString=[]  Role=Automatic
      settings: SourceProductName=Bose Talaria
  TrivialTranslation : TuneVar/TrivialTranslation  TriggerInit=[300 28 350 72]
      settings: SourceProductName=Bose Talaria
  Tune Variable : TuneVar/TuneVar  TuneName=RampTime  SpecifyMaxSize=off  VariableDim=1 (Row)  MaxSize=[1 1]  TunabilityNumber=1  MinValue=MinValue  MaxValue=MaxValue  TriggerInit=[20 25 190 75]  MaskValue=MaskValue
      settings: SourceProductName=Bose Talaria
  wires:
  TrivialTranslation/1 -> TOP/1
  Tune Variable/1 -> TrivialTranslation/1  "RampTime"

== system BasicAudio_TranslationEngine64/BasicAudio/Mute/mute/InnerLink/MuteControl/TuneVarRampTime ==
  TOP : TOP/TOP  TriggerInit=[440 20 585 80]  TopName=RampTime  DataTypeOut=single  BankNumber=BankNumber  PreOverlay=PreOverlay  PostOverlay=PostOverlay  CompatibilityString=[]  Role=Automatic
      settings: SourceProductName=Bose Talaria
  TrivialTranslation : TuneVar/TrivialTranslation  TriggerInit=[300 28 350 72]
      settings: SourceProductName=Bose Talaria
  Tune Variable : TuneVar/TuneVar  TuneName=RampTime  SpecifyMaxSize=off  VariableDim=1 (Row)  MaxSize=[1 1]  TunabilityNumber=1  MinValue=MinValue  MaxValue=MaxValue  TriggerInit=[20 25 190 75]  MaskValue=MaskValue
      settings: SourceProductName=Bose Talaria
  wires:
  Tune Variable/1 -> TrivialTranslation/1  "RampTime"
  TrivialTranslation/1 -> TOP/1

== system BasicAudio_TranslationEngine64/BasicAudio/Volume/volume/InnerLink/Index2DbTable/TuneTOP ==
  TOP : TOP/TOP  TriggerInit=[440 20 585 80]  TopName=maxgain  DataTypeOut=single  BankNumber=BankNumber  PreOverlay=PreOverlay  PostOverlay=PostOverlay  CompatibilityString=[]  Role=Automatic
      settings: SourceProductName=Bose Talaria
  TrivialTranslation : TuneVar/TrivialTranslation  TriggerInit=[300 28 350 72]
      settings: SourceProductName=Bose Talaria
  Tune Variable : TuneVar/TuneVar  TuneName=maxgain  SpecifyMaxSize=off  VariableDim=1 (Row)  MaxSize=[1 1]  TunabilityNumber=1  MinValue=MinValue  MaxValue=MaxValue  TriggerInit=[20 25 190 75]  MaskValue=MaskValue
      settings: SourceProductName=Bose Talaria
  wires:
  Tune Variable/1 -> TrivialTranslation/1  "maxgain"
  TrivialTranslation/1 -> TOP/1

== matlab function BasicAudio_TranslationEngine64/BasicAudio/Treble/Tone/InnerLink/tone filter tune translate4 ==
  data: maxOut output; maxIn input
  events: trigger input FUNCTION_CALL_EVENT
function maxOut  = fcn( ...
    maxIn) ... % inputs % parameters
%#codegen

% Just make sure the maximum is a positive dB value
maxOut = single(abs(maxIn.Value));

== matlab function BasicAudio_TranslationEngine64/BasicAudio/Volume/volume/InnerLink/Index2DbTable/table translation ==
  data: Table_Idx output; Table_dB output; Table input
  events: trigger input FUNCTION_CALL_EVENT
function [Table_Idx,Table_dB] = fcn(Table)
%#codegen
%
% Demux table matrix into one dimesional value and index vectors
%
%
% Set up the size and datatype of our TOP outputs:
maxTableSize = numel(Table.Value) / 2;
idxType = 'uint8';
idxStorageType = 'uint32';
dbType = 'single';
Table_Idx = zeros(1,maxTableSize,idxStorageType);
Table_dB = zeros(1,maxTableSize,dbType);

% separate the pairs into their index and value components
givenPairs = Table.Size(1);
indexes = Table.Value(1:givenPairs,1);
values = Table.Value(1:givenPairs,2);

% then sort and ignore duplicates
[cleanIdx,map] = unique(indexes);

% Validate input sizes
numPairs = numel(map);
argName='Table';

% Validate: enough data?
if (numPairs < 2)
    TranslateError('%s must have at least 2 index pairs. Encounted value with only %f pairs\n', argName, numPairs);
end

% Validate: Highest index still below 1.0?
if (cleanIdx(end) > 1)
    TranslateError('%s out of range table index %f encountered. Index must be between 0 and 1.\n',argName,cleanIdx(end));
end

% fill in the table buffer with provided pairs
for i=1:numPairs
    Table_Idx(i) = intmax(idxType) * cleanIdx(i);
    Table_dB(i) = values(map(i));
end
% fill the rest of the table buffer with the last entry
for j=numel(map)+1:maxTableSize
    Table_Idx(j) = Table_Idx(numPairs);
    Table_dB(j) =  Table_dB(numPairs);
end

end

== matlab function BasicAudio_TranslationEngine64/BasicAudio/Bass/Tone/InnerLink/tone filter tune translate1 ==
  data: FilterCoeffs output; FilterFrequencyHz input; Fs input; MaskFilterType parameter
  events: trigger input FUNCTION_CALL_EVENT
function FilterCoeffs  = fcn( ...
    FilterFrequencyHz, Fs, ... % inputs
    MaskFilterType ) % parameters
%#codegen

omega = 2 * pi * FilterFrequencyHz.Value / Fs;

A = (1 - sin(omega)) / cos(omega);

if (MaskFilterType == ToneMask.TypeLowpass)
    % lowpass coeffs (e.g. bass)
    B0 = (1 - A) / 2;
    B1 = B0;
else
    % highpass coeffs (e.g. treble)
    B0 = (1 + A) / 2;
    B1 = 0 - B0;
end

FilterCoeffs = single([B0 B1 A]);

== matlab function BasicAudio_TranslationEngine64/BasicAudio/Balance/balance/InnerLink/channel_ramper_translation ==
  data: ChanRampMap output; TuneChanRampMap input; channelCount input; MaskNumRampers parameter
  events: trigger input FUNCTION_CALL_EVENT
function ChanRampMap  = fcn(TuneChanRampMap, channelCount, ... % inputs
    MaskNumRampers) % parameters

% Verifies if each channel is assigned to one of the 4 possible rampers. 
% Acceptable rampers:
% 1: left
% 2: right
% 3: center
% 4: unused

argName = 'Balance';

% Ensure each channel is present in the map
inputMapWidth = numel(TuneChanRampMap.Value);
if (inputMapWidth ~= channelCount)
   error(['Error in %s : Channel-to-ramper map width [%d] does not match number of ',...
       'audio channels [%d]. Make sure all channels are assigned ',...
       'to either the left or right groups.'], argName, inputMapWidth, ...
       channelCount);
end

% Verify that the channels are assigned to valid group numbers.

if (numel(unique(TuneChanRampMap.Value)) > (MaskNumRampers + 1))
    error(['Error in [%s] : Atleast 1 channel has been assigned to the incorrect group.' ...
        'Group numbers assigned to channels in the Channel-to-ramper '...
        'map should be a number between 1 and 4, corresponding to one '...
        'of the 4 possible speaker contents .'], argName);        
end

if (sum(TuneChanRampMap.Value == 0) > 0)
   error(['Error in [%s] : Valid ramper values for the channel to '...
       'ramper map must be between 1 and 4, or "-1" to indicate an '... 
       'unused channel .'], argName);
end

ChanRampMap = int32(TuneChanRampMap.Value);

== matlab function BasicAudio_TranslationEngine64/BasicAudio/Treble/Tone/InnerLink/tone filter tune translate1 ==
  data: FilterCoeffs output; FilterFrequencyHz input; Fs input; MaskFilterType parameter
  events: trigger input FUNCTION_CALL_EVENT
function FilterCoeffs  = fcn( ...
    FilterFrequencyHz, Fs, ... % inputs
    MaskFilterType ) % parameters
%#codegen

omega = 2 * pi * FilterFrequencyHz.Value / Fs;

A = (1 - sin(omega)) / cos(omega);

if (MaskFilterType == ToneMask.TypeLowpass)
    % lowpass coeffs (e.g. bass)
    B0 = (1 - A) / 2;
    B1 = B0;
else
    % highpass coeffs (e.g. treble)
    B0 = (1 + A) / 2;
    B1 = 0 - B0;
end

FilterCoeffs = single([B0 B1 A]);

== matlab function BasicAudio_TranslationEngine64/BasicAudio/Balance/balance/InnerLink/TuneVarTable/Balance_Table_Translation ==
  data: tableDb output; tableIdx output; balanceTable input
  events: trigger input FUNCTION_CALL_EVENT
function [tableDb, tableIdx] = fcn(balanceTable)
%#codegen

% Set up the size and datatype of our TOP outputs:
maxTableSize = numel(balanceTable.Value) / 2;
idxType = 'uint8';
idxStorageType = 'uint32';
dbType = 'single';
tableIdx = zeros(1,maxTableSize,idxStorageType);
tableDb = zeros(1,maxTableSize,dbType);

% separate the pairs into their index and value components
givenPairs = balanceTable.Size(1);
indexes = balanceTable.Value(1:givenPairs,1);
values = balanceTable.Value(1:givenPairs,2);

% then sort and ignore duplicates
[cleanIdx,map] = unique(indexes);

% Validate input sizes
numPairs = numel(map);
argName='BalanceTable';

% Validate: enough data?
if (numPairs < 2)
    TranslateError('%s must have at least 2 index pairs. Encounted value with only %f pairs\n', argName, numPairs);
end

% Validate: Highest index still below 255?
if (cleanIdx(1) < 0 || cleanIdx(end) > intmax(idxType))
    TranslateError('%s out of range table index %f encountered. Index must be between 0 and %d.\n',argName,cleanIdx(end),intmax(idxType));
end

% fill in the table buffer with provided pairs
tableIdx(1:numPairs) = cleanIdx(1:numPairs);
tableDb(1:numPairs) = values(map(1:numPairs));

% fill the rest of the table buffer with the last entry
remainingPairs = numel(map)+1:maxTableSize;
tableIdx(remainingPairs) = tableIdx(numPairs);
tableDb(remainingPairs) =  tableDb(numPairs);

end

== matlab function BasicAudio_TranslationEngine64/BasicAudio/Bass/Tone/InnerLink/tone filter tune translate2 ==
  data: FilterCoeffs output; FilterFrequencyHz input; Fs input; MaskFilterType parameter
  events: trigger input FUNCTION_CALL_EVENT
function FilterCoeffs  = fcn( ...
    FilterFrequencyHz, Fs, ... % inputs
    MaskFilterType ) % parameters
%#codegen

omega = 2 * pi * FilterFrequencyHz.Value / Fs;

A = (1 - sin(omega)) / cos(omega);

if (MaskFilterType == ToneMask.TypeLowpass)
    % lowpass coeffs (e.g. bass)
    B0 = (1 - A) / 2;
    B1 = B0;
else
    % highpass coeffs (e.g. treble)
    B0 = (1 + A) / 2;
    B1 = 0 - B0;
end

FilterCoeffs = single([B0 B1 A]);
